simulink model "state_feedback_controller"  (R2024a)
settings: Solver=VariableStepAuto  StartTime=0.0  StopTime=10.0  RelTol=1e-3
undefined symbols (not defined in the file): b, J, K, Kc, L, Nbar, R
settings Model: Creator=Harish  LastModifiedBy=Harish

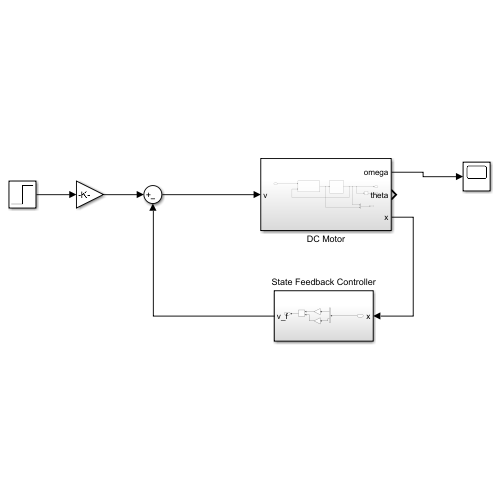
[thumbnail: Simulink's stored preview of the top-level diagram]
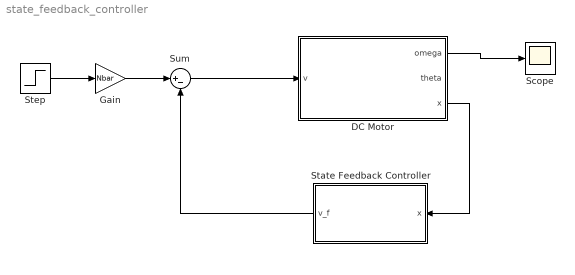
== system state_feedback_controller ==
  DC Motor : Subsystem
  Gain : Gain  Gain=Nbar
  Scope : Scope
  State Feedback Controller : Subsystem
  Step : Step  SampleTime=0
  Sum : Sum  Inputs=|+-
  wires:
  Sum/1 -> DC Motor/1(v)
  DC Motor/1(omega) -> Scope/1
  DC Motor/3(x) -> State Feedback Controller/1(x)
  Step/1 -> Gain/1
  State Feedback Controller/1(v_f) -> Sum/2
  Gain/1 -> Sum/1

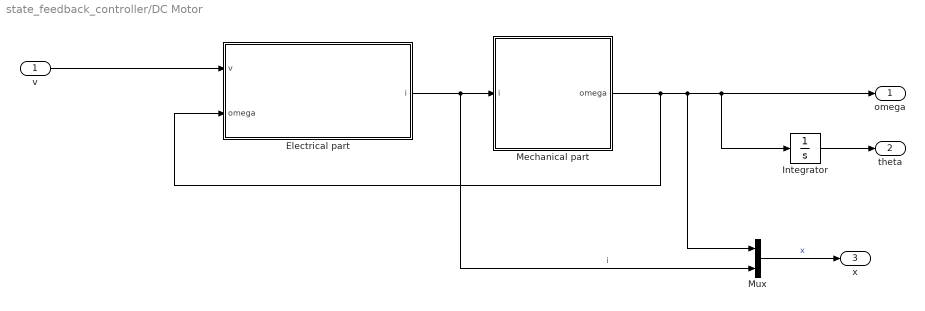
== system state_feedback_controller/DC Motor ==
  v : Inport
  "Electrical part " : Subsystem
  Integrator : Integrator
  Mechanical part : Subsystem
  Mux : Mux  Inputs=2
  omega : Outport
  theta : Outport  Port=2
  x : Outport  Port=3
  wires:
  "Electrical part "/1(i) -> Mux/2, Mechanical part/1(i)  "i"
  Mechanical part/1(omega) -> Mux/1, Integrator/1, omega/1, "Electrical part "/2(omega)
  v/1 -> "Electrical part "/1(v)
  Integrator/1 -> theta/1
  Mux/1 -> x/1  "x"

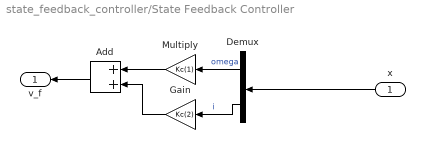
== system state_feedback_controller/State Feedback Controller ==
  x : Inport
  Add : Sum
  Demux : Demux  Outputs=2
  Gain : Gain  Gain=Kc(2)
  Multiply : Gain  Gain=Kc(1)
  v_f : Outport
  wires:
  x/1 -> Demux/1
  Multiply/1 -> Add/1
  Add/1 -> v_f/1
  Demux/1 -> Multiply/1  "omega"
  Demux/2 -> Gain/1  "i"
  Gain/1 -> Add/2

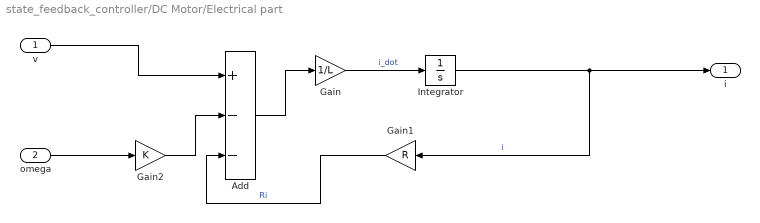
== system state_feedback_controller/DC Motor/Electrical part  ==
  v : Inport
  omega : Inport  Port=2
  Add : Sum  Inputs=+--
  Gain : Gain  Gain=1/L
  Gain1 : Gain  Gain=R
  Gain2 : Gain  Gain=K
  Integrator : Integrator
  i : Outport
  wires:
  Add/1 -> Gain/1
  Integrator/1 -> i/1, Gain1/1  "i"
  Gain1/1 -> Add/3  "Ri"
  v/1 -> Add/1
  Gain2/1 -> Add/2
  Gain/1 -> Integrator/1  "i_dot"
  omega/1 -> Gain2/1

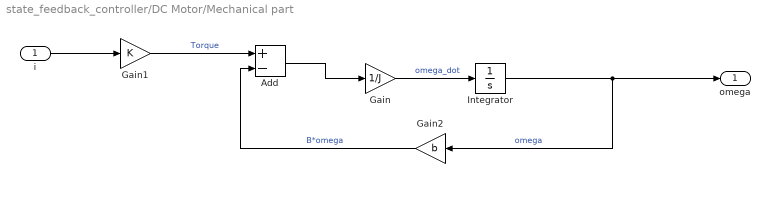
== system state_feedback_controller/DC Motor/Mechanical part ==
  i : Inport
  Add : Sum  Inputs=+-
  Gain : Gain  Gain=1/J
  Gain1 : Gain  Gain=K
  Gain2 : Gain  Gain=b
  Integrator : Integrator
  omega : Outport
  wires:
  Add/1 -> Gain/1
  Integrator/1 -> omega/1, Gain2/1  "omega"
  Gain2/1 -> Add/2  "B*omega"
  i/1 -> Gain1/1
  Gain/1 -> Integrator/1  "omega_dot"
  Gain1/1 -> Add/1  "Torque"
